simulink library "LIB_InputsProcessing"  (R2018b)
settings: Solver=VariableStepAuto  StartTime=0.0  StopTime=10.0  RelTol=1e-3
undefined symbols (not defined in the file or in its folder): rTBlowerMotorMeasuredFilter, rVBatteryMeasuredFilter, TBlowerMotorScaledValueMap, VAnalogInputSpan, VTBlowerMotorScaledValueAxis
libraries: RespiratorCtrlLib x11
settings Model: Creator=BRAUL  LastModifiedBy=VITIE

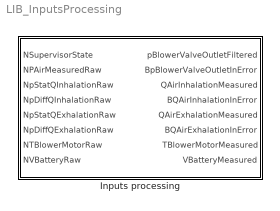
== system LIB_InputsProcessing ==
  Inputs processing : Subsystem
      settings: AttributesFormatString=%<ReferenceBlock>

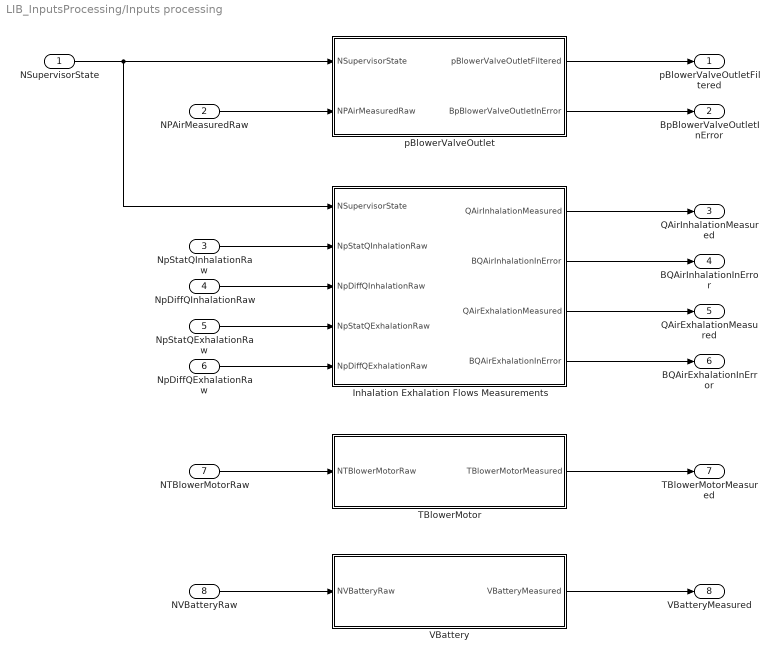
== system LIB_InputsProcessing/Inputs processing ==
  NSupervisorState : Inport  OutDataTypeStr=Enum: eSupervisorStates
  NPAirMeasuredRaw : Inport  Port=2
  NpStatQInhalationRaw : Inport  Port=3  OutDataTypeStr=single
  NpDiffQInhalationRaw : Inport  Port=4  OutDataTypeStr=single
  NpStatQExhalationRaw : Inport  Port=5  OutDataTypeStr=single
  NpDiffQExhalationRaw : Inport  Port=6  OutDataTypeStr=single
  NTBlowerMotorRaw : Inport  Port=7
  NVBatteryRaw : Inport  Port=8
  Inhalation Exhalation Flows Measurements : Subsystem
  TBlowerMotor : Subsystem
  VBattery : Subsystem
  pBlowerValveOutlet : Subsystem
  pBlowerValveOutletFiltered : Outport
  BpBlowerValveOutletInError : Outport  Port=2  OutDataTypeStr=boolean
  QAirInhalationMeasured : Outport  Port=3  OutDataTypeStr=single
  BQAirInhalationInError : Outport  Port=4  OutDataTypeStr=boolean
  QAirExhalationMeasured : Outport  Port=5  OutDataTypeStr=single
  BQAirExhalationInError : Outport  Port=6  OutDataTypeStr=boolean
  TBlowerMotorMeasured : Outport  Port=7
  VBatteryMeasured : Outport  Port=8
  wires:
  Inhalation Exhalation Flows Measurements/4(BQAirExhalationInError) -> BQAirExhalationInError/1
  Inhalation Exhalation Flows Measurements/3(QAirExhalationMeasured) -> QAirExhalationMeasured/1
  Inhalation Exhalation Flows Measurements/2(BQAirInhalationInError) -> BQAirInhalationInError/1
  Inhalation Exhalation Flows Measurements/1(QAirInhalationMeasured) -> QAirInhalationMeasured/1
  NpDiffQExhalationRaw/1 -> Inhalation Exhalation Flows Measurements/5(NpDiffQExhalationRaw)
  NpStatQExhalationRaw/1 -> Inhalation Exhalation Flows Measurements/4(NpStatQExhalationRaw)
  NpDiffQInhalationRaw/1 -> Inhalation Exhalation Flows Measurements/3(NpDiffQInhalationRaw)
  NpStatQInhalationRaw/1 -> Inhalation Exhalation Flows Measurements/2(NpStatQInhalationRaw)
  pBlowerValveOutlet/1(pBlowerValveOutletFiltered) -> pBlowerValveOutletFiltered/1
  pBlowerValveOutlet/2(BpBlowerValveOutletInError) -> BpBlowerValveOutletInError/1
  NSupervisorState/1 -> pBlowerValveOutlet/1(NSupervisorState), Inhalation Exhalation Flows Measurements/1(NSupervisorState)
  NPAirMeasuredRaw/1 -> pBlowerValveOutlet/2(NPAirMeasuredRaw)
  VBattery/1(VBatteryMeasured) -> VBatteryMeasured/1
  TBlowerMotor/1(TBlowerMotorMeasured) -> TBlowerMotorMeasured/1
  NVBatteryRaw/1 -> VBattery/1(NVBatteryRaw)
  NTBlowerMotorRaw/1 -> TBlowerMotor/1(NTBlowerMotorRaw)

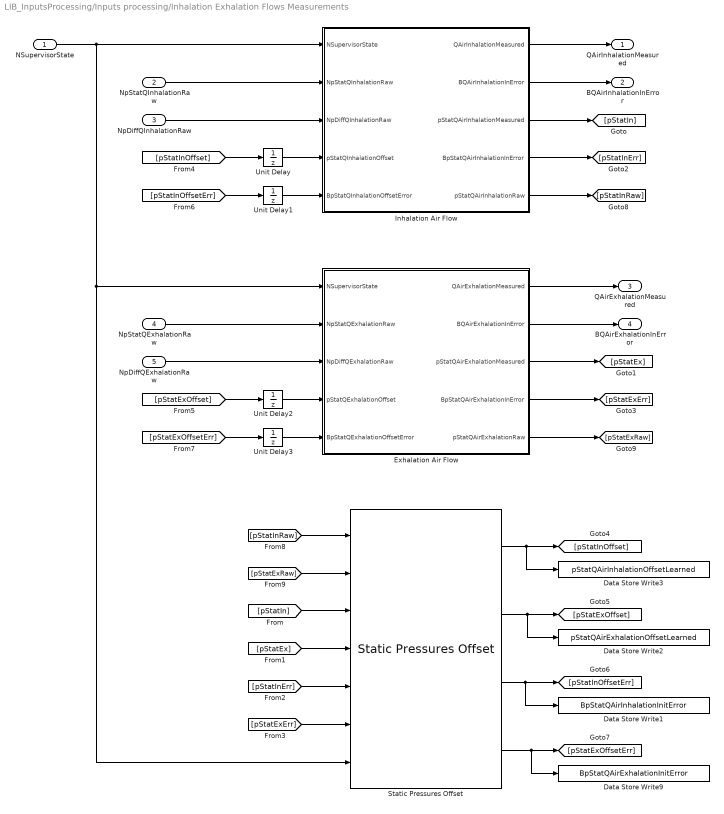
== system LIB_InputsProcessing/Inputs processing/Inhalation Exhalation Flows Measurements ==
  NSupervisorState : Inport  OutDataTypeStr=Enum: eSupervisorStates
  NpStatQInhalationRaw : Inport  Port=2  OutDataTypeStr=single
  NpDiffQInhalationRaw : Inport  Port=3  OutDataTypeStr=single
  NpStatQExhalationRaw : Inport  Port=4  OutDataTypeStr=single
  NpDiffQExhalationRaw : Inport  Port=5  OutDataTypeStr=single
  Data Store Write1 : DataStoreWrite  DataStoreName=BpStatQAirInhalationInitError
  Data Store Write2 : DataStoreWrite  DataStoreName=pStatQAirExhalationOffsetLearned
  Data Store Write3 : DataStoreWrite  DataStoreName=pStatQAirInhalationOffsetLearned
  Data Store Write9 : DataStoreWrite  DataStoreName=BpStatQAirExhalationInitError
  Exhalation Air Flow : Subsystem
  Inhalation Air Flow : Subsystem
  Static Pressures Offset : RespiratorCtrlLib/Inputs/Static Pressures Offset  pOffsetMin=pStatQAirAutoOffsetMin  pOffsetMax=pStatQAirAutoOffsetMax  pOffsetRateMax=pStatQAirAutoOffsetRateMax
  Unit Delay{,1..3} (4 alike) : UnitDelay  SampleTime=-1
  QAirInhalationMeasured : Outport  OutDataTypeStr=single
  BQAirInhalationInError : Outport  Port=2  OutDataTypeStr=boolean
  QAirExhalationMeasured : Outport  Port=3  OutDataTypeStr=single
  BQAirExhalationInError : Outport  Port=4  OutDataTypeStr=boolean
  wires:
  [pStatExRaw] -> Static Pressures Offset/2
  [pStatInRaw] -> Static Pressures Offset/1
  Exhalation Air Flow/5(pStatQAirExhalationRaw) -> [pStatExRaw]
  Inhalation Air Flow/5(pStatQAirInhalationRaw) -> [pStatInRaw]
  [pStatExOffsetErr] -> Unit Delay3/1
  [pStatExOffset] -> Unit Delay2/1
  Unit Delay3/1 -> Exhalation Air Flow/5(BpStatQExhalationOffsetError)
  Unit Delay2/1 -> Exhalation Air Flow/4(pStatQExhalationOffset)
  [pStatInOffsetErr] -> Unit Delay1/1
  [pStatInOffset] -> Unit Delay/1
  Unit Delay1/1 -> Inhalation Air Flow/5(BpStatQInhalationOffsetError)
  Unit Delay/1 -> Inhalation Air Flow/4(pStatQInhalationOffset)
  Static Pressures Offset/4 -> [pStatExOffsetErr], Data Store Write9/1
  Static Pressures Offset/3 -> [pStatInOffsetErr], Data Store Write1/1
  Static Pressures Offset/2 -> [pStatExOffset], Data Store Write2/1
  Static Pressures Offset/1 -> [pStatInOffset], Data Store Write3/1
  [pStatExErr] -> Static Pressures Offset/6
  [pStatInErr] -> Static Pressures Offset/5
  [pStatEx] -> Static Pressures Offset/4
  [pStatIn] -> Static Pressures Offset/3
  Exhalation Air Flow/4(BpStatQAirExhalationInError) -> [pStatExErr]
  Inhalation Air Flow/4(BpStatQAirInhalationInError) -> [pStatInErr]
  Exhalation Air Flow/3(pStatQAirExhalationMeasured) -> [pStatEx]
  Inhalation Air Flow/3(pStatQAirInhalationMeasured) -> [pStatIn]
  NSupervisorState/1 -> Exhalation Air Flow/1(NSupervisorState), Static Pressures Offset/7, Inhalation Air Flow/1(NSupervisorState)
  Exhalation Air Flow/2(BQAirExhalationInError) -> BQAirExhalationInError/1
  Exhalation Air Flow/1(QAirExhalationMeasured) -> QAirExhalationMeasured/1
  Inhalation Air Flow/2(BQAirInhalationInError) -> BQAirInhalationInError/1
  Inhalation Air Flow/1(QAirInhalationMeasured) -> QAirInhalationMeasured/1
  NpDiffQExhalationRaw/1 -> Exhalation Air Flow/3(NpDiffQExhalationRaw)
  NpStatQExhalationRaw/1 -> Exhalation Air Flow/2(NpStatQExhalationRaw)
  NpDiffQInhalationRaw/1 -> Inhalation Air Flow/3(NpDiffQInhalationRaw)
  NpStatQInhalationRaw/1 -> Inhalation Air Flow/2(NpStatQInhalationRaw)

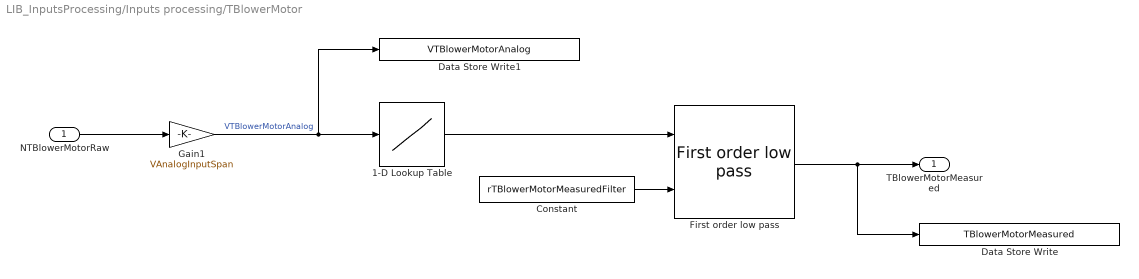
== system LIB_InputsProcessing/Inputs processing/TBlowerMotor ==
  NTBlowerMotorRaw : Inport
  1-D Lookup Table : Lookup_n-D  NumberOfTableDimensions=1  BreakpointsForDimension1=VTBlowerMotorScaledValueAxis  BeginIndexSearchUsingPreviousIndexResult=on  Table=TBlowerMotorScaledValueMap  ExtrapMethod=Clip  RemoveProtectionInput=on  UseLastTableValue=on  InternalRulePriority=Speed  RndMeth=Simplest  InputSameDT=on
  Constant : Constant  Value=rTBlowerMotorMeasuredFilter
  Data Store Write : DataStoreWrite  DataStoreName=TBlowerMotorMeasured
  Data Store Write1 : DataStoreWrite  DataStoreName=VTBlowerMotorAnalog
  First order low pass : RespiratorCtrlLib/Filters/First order low pass  SystemSampleTime=-1
  Gain1 : Gain  Gain=VAnalogInputSpan
      settings: AttributesFormatString=%<Gain>
  TBlowerMotorMeasured : Outport
  wires:
  Constant/1 -> First order low pass/2
  1-D Lookup Table/1 -> First order low pass/1
  Gain1/1 -> 1-D Lookup Table/1, Data Store Write1/1  "VTBlowerMotorAnalog"
  First order low pass/1 -> TBlowerMotorMeasured/1, Data Store Write/1
  NTBlowerMotorRaw/1 -> Gain1/1

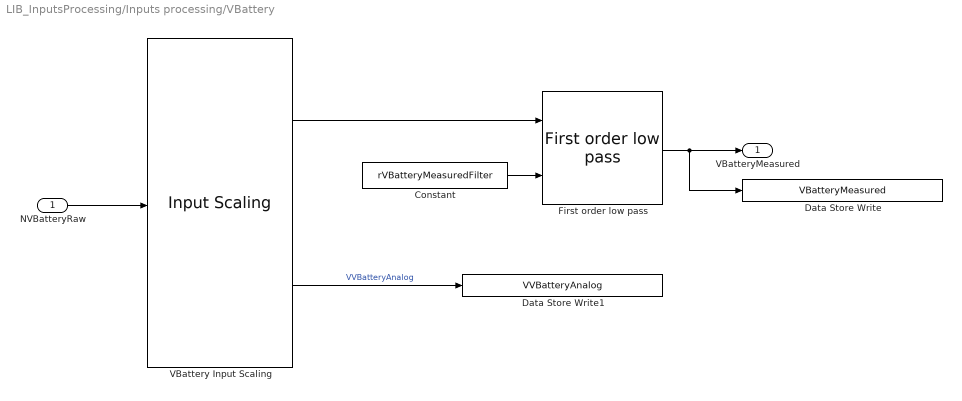
== system LIB_InputsProcessing/Inputs processing/VBattery ==
  NVBatteryRaw : Inport
  Constant : Constant  Value=rVBatteryMeasuredFilter
  Data Store Write : DataStoreWrite  DataStoreName=VBatteryMeasured
  Data Store Write1 : DataStoreWrite  DataStoreName=VVBatteryAnalog
  First order low pass : RespiratorCtrlLib/Filters/First order low pass  SystemSampleTime=-1
  VBattery Input Scaling : RespiratorCtrlLib/Inputs/Input Scaling  inputName=VBattery  elecMin=VVBatteryAnalogMin  elecMax=VVBatteryAnalogMax  physicMin=VBatteryMeasuredScaleMin  physicMax=VBatteryMeasuredScaleMax  gain=0  offset=0
  VBatteryMeasured : Outport
  wires:
  NVBatteryRaw/1 -> VBattery Input Scaling/1
  VBattery Input Scaling/2 -> Data Store Write1/1  "VVBatteryAnalog"
  First order low pass/1 -> VBatteryMeasured/1, Data Store Write/1
  VBattery Input Scaling/1 -> First order low pass/1
  Constant/1 -> First order low pass/2

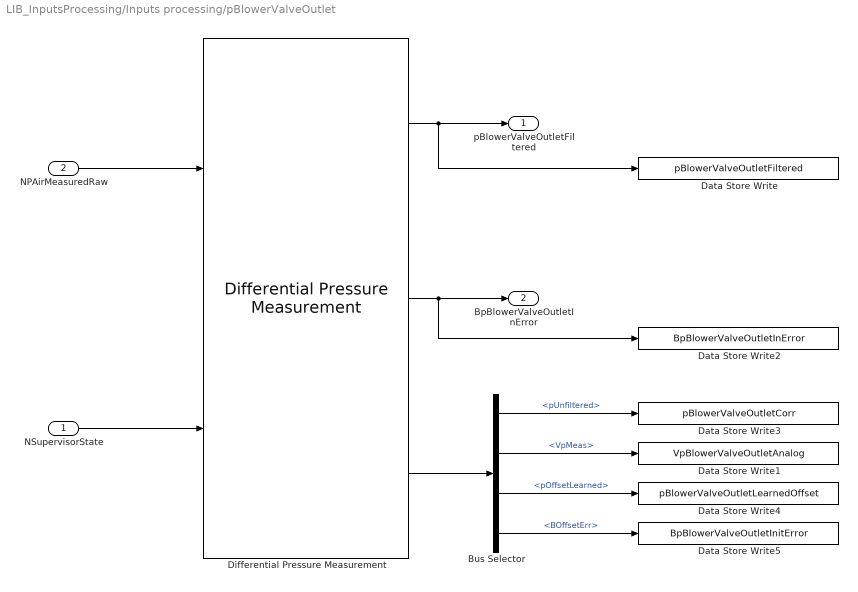
== system LIB_InputsProcessing/Inputs processing/pBlowerValveOutlet ==
  NSupervisorState : Inport  OutDataTypeStr=Enum: eSupervisorStates
  NPAirMeasuredRaw : Inport  Port=2
  Bus Selector : BusSelector  OutputSignals=pUnfiltered,VpMeas,pOffsetLearned,BOffsetErr
  Data Store Write : DataStoreWrite  DataStoreName=pBlowerValveOutletFiltered
  Data Store Write1 : DataStoreWrite  DataStoreName=VpBlowerValveOutletAnalog
  Data Store Write2 : DataStoreWrite  DataStoreName=BpBlowerValveOutletInError
  Data Store Write3 : DataStoreWrite  DataStoreName=pBlowerValveOutletCorr
  Data Store Write4 : DataStoreWrite  DataStoreName=pBlowerValveOutletLearnedOffset
  Data Store Write5 : DataStoreWrite  DataStoreName=BpBlowerValveOutletInitError
  Differential Pressure Measurement : RespiratorCtrlLib/Inputs/Differential Pressure Measurement  MeasName=pBlowerValveOutlet  AnalogMin=VpBlowerValveOutletAnalogMin  AnalogMax=VpBlowerValveOutletAnalogMax  PressureMin=pBlowerValveOutletScaledMin  PressureMax=pBlowerValveOutletScaledMax  ZeroOffset=pBlowerValveOutletMeasureOffset  CutOffFreq=fpBlowerValveOutletFilter  pOffsetMin=pBlowerValveOutletOffsetMin  pOffsetMax=pBlowerValveOutletOffsetMax  pOffsetRateMax=pBlowerValveOutletOffsetRateMax  VAnaMinDiag=VpBlowerValveOutletAnalogDiagMin  VAnaMaxDiag=VpBlowerValveOutletAnalogDiagMax
  pBlowerValveOutletFiltered : Outport
  BpBlowerValveOutletInError : Outport  Port=2  OutDataTypeStr=boolean
  wires:
  Bus Selector/4 -> Data Store Write5/1  "<BOffsetErr>"
  Bus Selector/3 -> Data Store Write4/1  "<pOffsetLearned>"
  Bus Selector/1 -> Data Store Write3/1  "<pUnfiltered>"
  Bus Selector/2 -> Data Store Write1/1  "<VpMeas>"
  Differential Pressure Measurement/3 -> Bus Selector/1
  NSupervisorState/1 -> Differential Pressure Measurement/2
  NPAirMeasuredRaw/1 -> Differential Pressure Measurement/1
  Differential Pressure Measurement/2 -> BpBlowerValveOutletInError/1, Data Store Write2/1
  Differential Pressure Measurement/1 -> pBlowerValveOutletFiltered/1, Data Store Write/1

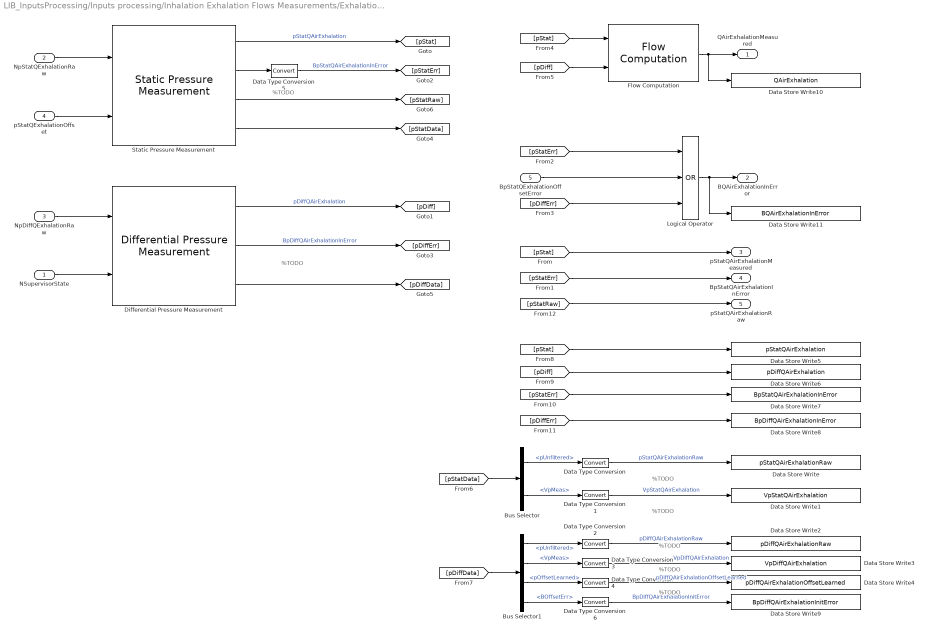
== system LIB_InputsProcessing/Inputs processing/Inhalation Exhalation Flows Measurements/Exhalation Air Flow ==
  note: %TODO
  note: %TODO
  note: %TODO
  note: %TODO
  note: %TODO
  note: %TODO
  note: %TODO
  NSupervisorState : Inport  OutDataTypeStr=Enum: eSupervisorStates
  NpStatQExhalationRaw : Inport  Port=2  OutDataTypeStr=single
  NpDiffQExhalationRaw : Inport  Port=3  OutDataTypeStr=single
  pStatQExhalationOffset : Inport  Port=4  OutDataTypeStr=single
  BpStatQExhalationOffsetError : Inport  Port=5  OutDataTypeStr=boolean
  Bus Selector : BusSelector  OutputSignals=pUnfiltered,VpMeas
  Bus Selector1 : BusSelector  OutputSignals=pUnfiltered,VpMeas,pOffsetLearned,BOffsetErr
  Data Store Write : DataStoreWrite  DataStoreName=pStatQAirExhalationRaw
  Data Store Write1 : DataStoreWrite  DataStoreName=VpStatQAirExhalation
  Data Store Write10 : DataStoreWrite  DataStoreName=QAirExhalation
  Data Store Write11 : DataStoreWrite  DataStoreName=BQAirExhalationInError
  Data Store Write2 : DataStoreWrite  DataStoreName=pDiffQAirExhalationRaw
  Data Store Write3 : DataStoreWrite  DataStoreName=VpDiffQAirExhalation
  Data Store Write4 : DataStoreWrite  DataStoreName=pDiffQAirExhalationOffsetLearned
  Data Store Write5 : DataStoreWrite  DataStoreName=pStatQAirExhalation
  Data Store Write6 : DataStoreWrite  DataStoreName=pDiffQAirExhalation
  Data Store Write7 : DataStoreWrite  DataStoreName=BpStatQAirExhalationInError
  Data Store Write8 : DataStoreWrite  DataStoreName=BpDiffQAirExhalationInError
  Data Store Write9 : DataStoreWrite  DataStoreName=BpDiffQAirExhalationInitError
  Data Type Conversion{,1..6} (7 alike) : DataTypeConversion
  Differential Pressure Measurement : RespiratorCtrlLib/Inputs/Differential Pressure Measurement  MeasName=Exhalation differential pressure  AnalogMin=VpDiffQAirAnalogicMin  AnalogMax=VpDiffQAirAnalogicMax  PressureMin=pDiffQAirScaledMax  PressureMax=pDiffQAirScaledMin  ZeroOffset=pDiffQAirExhalationOffset  CutOffFreq=fpDiffQAirExhalation  pOffsetMin=pDiffQAirAutoOffsetMin  pOffsetMax=pDiffQAirAutoOffsetMax  pOffsetRateMax=pDiffQAirAutoOffsetRateMax  VAnaMinDiag=VpDiffQAirAnalogicDiagMin  VAnaMaxDiag=VpDiffQAirAnalogicDiagMax
  Flow Computation : RespiratorCtrlLib/Inputs/Flow Computation  measName=Exhalation  QRef=QExhalationReference  PStatRef=pStaticQExhalationReference  PDiffRef=pDifferentialQExhalationReference  kAlpha=kAlphaQExhalation  kBeta=kBetaQExhalation
  Logical Operator : Logic  Operator=OR  Inputs=3  AllPortsSameDT=off  OutDataTypeStr=boolean
  Static Pressure Measurement : RespiratorCtrlLib/Inputs/Static Pressure Measurement  MeasName=Exhalation static pressure  AnalogMin=VpStatQAirAnalogicMin  AnalogMax=VpStatQAirAnalogicMax  PressureMin=pStatQAirScaledMin  PressureMax=pStatQAirScaledMax  ZeroOffset=pStatQAirExhalationOffset  CutOffFreq=fpStatQAirExhalation  VAnaMinDiag=VpStatQAirAnalogicDiagMin  VAnaMaxDiag=VpStatQAirAnalogicDiagMax
  QAirExhalationMeasured : Outport  OutDataTypeStr=single
  BQAirExhalationInError : Outport  Port=2  OutDataTypeStr=boolean
  pStatQAirExhalationMeasured : Outport  Port=3  OutDataTypeStr=single
  BpStatQAirExhalationInError : Outport  Port=4  OutDataTypeStr=boolean
  pStatQAirExhalationRaw : Outport  Port=5  OutDataTypeStr=single
  wires:
  [pStatRaw] -> pStatQAirExhalationRaw/1
  Static Pressure Measurement/3 -> [pStatRaw]
  Static Pressure Measurement/4 -> [pStatData]
  Data Type Conversion6/1 -> Data Store Write9/1  "BpDiffQAirExhalationInitError"
  Bus Selector1/4 -> Data Type Conversion6/1  "<BOffsetErr>"
  Data Type Conversion5/1 -> [pStatErr]  "BpStatQAirExhalationInError"
  [pStatData] -> Bus Selector/1
  [pDiffData] -> Bus Selector1/1
  Bus Selector/1 -> Data Type Conversion/1  "<pUnfiltered>"
  Bus Selector/2 -> Data Type Conversion1/1  "<VpMeas>"
  Bus Selector1/1 -> Data Type Conversion2/1  "<pUnfiltered>"
  Bus Selector1/2 -> Data Type Conversion3/1  "<VpMeas>"
  Bus Selector1/3 -> Data Type Conversion4/1  "<pOffsetLearned>"
  Data Type Conversion/1 -> Data Store Write/1  "pStatQAirExhalationRaw"
  Data Type Conversion1/1 -> Data Store Write1/1  "VpStatQAirExhalation"
  Data Type Conversion2/1 -> Data Store Write2/1  "pDiffQAirExhalationRaw"
  Data Type Conversion3/1 -> Data Store Write3/1  "VpDiffQAirExhalation"
  Data Type Conversion4/1 -> Data Store Write4/1  "pDiffQAirExhalationOffsetLearned"
  [pStat] -> Data Store Write5/1
  [pDiff] -> Data Store Write6/1
  [pStatErr] -> Data Store Write7/1
  [pDiffErr] -> Data Store Write8/1
  NSupervisorState/1 -> Differential Pressure Measurement/2
  NpDiffQExhalationRaw/1 -> Differential Pressure Measurement/1
  pStatQExhalationOffset/1 -> Static Pressure Measurement/2
  NpStatQExhalationRaw/1 -> Static Pressure Measurement/1
  [pDiffErr] -> Logical Operator/3
  Differential Pressure Measurement/3 -> [pDiffData]
  Differential Pressure Measurement/1 -> [pDiff]  "pDiffQAirExhalation"
  Static Pressure Measurement/1 -> [pStat]  "pStatQAirExhalation"
  Differential Pressure Measurement/2 -> [pDiffErr]  "BpDiffQAirExhalationInError"
  [pStatErr] -> Logical Operator/1
  Logical Operator/1 -> BQAirExhalationInError/1, Data Store Write11/1
  [pStat] -> pStatQAirExhalationMeasured/1
  BpStatQExhalationOffsetError/1 -> Logical Operator/2
  [pStat] -> Flow Computation/1
  Flow Computation/1 -> QAirExhalationMeasured/1, Data Store Write10/1
  [pDiff] -> Flow Computation/2
  Static Pressure Measurement/2 -> Data Type Conversion5/1
  [pStatErr] -> BpStatQAirExhalationInError/1

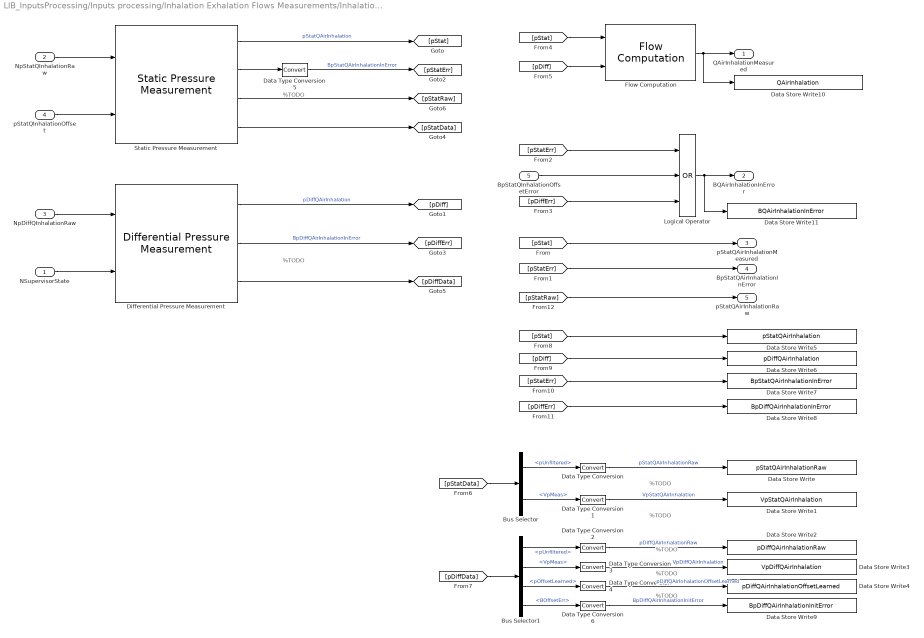
== system LIB_InputsProcessing/Inputs processing/Inhalation Exhalation Flows Measurements/Inhalation Air Flow ==
  note: %TODO
  note: %TODO
  note: %TODO
  note: %TODO
  note: %TODO
  note: %TODO
  note: %TODO
  NSupervisorState : Inport  OutDataTypeStr=Enum: eSupervisorStates
  NpStatQInhalationRaw : Inport  Port=2  OutDataTypeStr=single
  NpDiffQInhalationRaw : Inport  Port=3  OutDataTypeStr=single
  pStatQInhalationOffset : Inport  Port=4  OutDataTypeStr=single
  BpStatQInhalationOffsetError : Inport  Port=5  OutDataTypeStr=boolean
  Bus Selector : BusSelector  OutputSignals=pUnfiltered,VpMeas
  Bus Selector1 : BusSelector  OutputSignals=pUnfiltered,VpMeas,pOffsetLearned,BOffsetErr
  Data Store Write : DataStoreWrite  DataStoreName=pStatQAirInhalationRaw
  Data Store Write1 : DataStoreWrite  DataStoreName=VpStatQAirInhalation
  Data Store Write10 : DataStoreWrite  DataStoreName=QAirInhalation
  Data Store Write11 : DataStoreWrite  DataStoreName=BQAirInhalationInError
  Data Store Write2 : DataStoreWrite  DataStoreName=pDiffQAirInhalationRaw
  Data Store Write3 : DataStoreWrite  DataStoreName=VpDiffQAirInhalation
  Data Store Write4 : DataStoreWrite  DataStoreName=pDiffQAirInhalationOffsetLearned
  Data Store Write5 : DataStoreWrite  DataStoreName=pStatQAirInhalation
  Data Store Write6 : DataStoreWrite  DataStoreName=pDiffQAirInhalation
  Data Store Write7 : DataStoreWrite  DataStoreName=BpStatQAirInhalationInError
  Data Store Write8 : DataStoreWrite  DataStoreName=BpDiffQAirInhalationInError
  Data Store Write9 : DataStoreWrite  DataStoreName=BpDiffQAirInhalationInitError
  Data Type Conversion{,1..6} (7 alike) : DataTypeConversion
  Differential Pressure Measurement : RespiratorCtrlLib/Inputs/Differential Pressure Measurement  MeasName=Inhalation differential pressure  AnalogMin=VpDiffQAirAnalogicMin  AnalogMax=VpDiffQAirAnalogicMax  PressureMin=pDiffQAirScaledMax  PressureMax=pDiffQAirScaledMin  ZeroOffset=pDiffQAirInhalationOffset  CutOffFreq=fpDiffQAirInhalation  pOffsetMin=pDiffQAirAutoOffsetMin  pOffsetMax=pDiffQAirAutoOffsetMax  pOffsetRateMax=pDiffQAirAutoOffsetRateMax  VAnaMinDiag=VpDiffQAirAnalogicDiagMin  VAnaMaxDiag=VpDiffQAirAnalogicDiagMax
  Flow Computation : RespiratorCtrlLib/Inputs/Flow Computation  measName=Inhalation  QRef=QInhalationReference  PStatRef=pStaticQInhalationReference  PDiffRef=pDifferentialQInhalationReference  kAlpha=kAlphaQInhalation  kBeta=kBetaQInhalation
  Logical Operator : Logic  Operator=OR  Inputs=3  AllPortsSameDT=off  OutDataTypeStr=boolean
  Static Pressure Measurement : RespiratorCtrlLib/Inputs/Static Pressure Measurement  MeasName=Inhalation static pressure  AnalogMin=VpStatQAirAnalogicMin  AnalogMax=VpStatQAirAnalogicMax  PressureMin=pStatQAirScaledMin  PressureMax=pStatQAirScaledMax  ZeroOffset=pStatQAirInhalationOffset  CutOffFreq=fpStatQAirInhalation  VAnaMinDiag=VpStatQAirAnalogicDiagMin  VAnaMaxDiag=VpStatQAirAnalogicDiagMax
  QAirInhalationMeasured : Outport  OutDataTypeStr=single
  BQAirInhalationInError : Outport  Port=2  OutDataTypeStr=boolean
  pStatQAirInhalationMeasured : Outport  Port=3  OutDataTypeStr=single
  BpStatQAirInhalationInError : Outport  Port=4  OutDataTypeStr=boolean
  pStatQAirInhalationRaw : Outport  Port=5  OutDataTypeStr=single
  wires:
  [pStatRaw] -> pStatQAirInhalationRaw/1
  Static Pressure Measurement/3 -> [pStatRaw]
  Data Type Conversion6/1 -> Data Store Write9/1  "BpDiffQAirInhalationInitError"
  Bus Selector1/4 -> Data Type Conversion6/1  "<BOffsetErr>"
  Data Type Conversion5/1 -> [pStatErr]  "BpStatQAirInhalationInError"
  [pDiffErr] -> Data Store Write8/1
  [pStatErr] -> Data Store Write7/1
  [pDiff] -> Data Store Write6/1
  [pStat] -> Data Store Write5/1
  Data Type Conversion4/1 -> Data Store Write4/1  "pDiffQAirInhalationOffsetLearned"
  Data Type Conversion3/1 -> Data Store Write3/1  "VpDiffQAirInhalation"
  Data Type Conversion2/1 -> Data Store Write2/1  "pDiffQAirInhalationRaw"
  Data Type Conversion1/1 -> Data Store Write1/1  "VpStatQAirInhalation"
  Data Type Conversion/1 -> Data Store Write/1  "pStatQAirInhalationRaw"
  Bus Selector1/3 -> Data Type Conversion4/1  "<pOffsetLearned>"
  Bus Selector1/2 -> Data Type Conversion3/1  "<VpMeas>"
  Bus Selector1/1 -> Data Type Conversion2/1  "<pUnfiltered>"
  Bus Selector/2 -> Data Type Conversion1/1  "<VpMeas>"
  Bus Selector/1 -> Data Type Conversion/1  "<pUnfiltered>"
  [pDiffData] -> Bus Selector1/1
  [pStatData] -> Bus Selector/1
  [pDiff] -> Flow Computation/2
  [pStat] -> Flow Computation/1
  Flow Computation/1 -> QAirInhalationMeasured/1, Data Store Write10/1
  [pDiffErr] -> Logical Operator/3
  BpStatQInhalationOffsetError/1 -> Logical Operator/2
  [pStatErr] -> Logical Operator/1
  Logical Operator/1 -> BQAirInhalationInError/1, Data Store Write11/1
  [pStat] -> pStatQAirInhalationMeasured/1
  [pStatErr] -> BpStatQAirInhalationInError/1
  Differential Pressure Measurement/3 -> [pDiffData]
  Static Pressure Measurement/4 -> [pStatData]
  Differential Pressure Measurement/2 -> [pDiffErr]  "BpDiffQAirInhalationInError"
  Static Pressure Measurement/2 -> Data Type Conversion5/1
  Differential Pressure Measurement/1 -> [pDiff]  "pDiffQAirInhalation"
  Static Pressure Measurement/1 -> [pStat]  "pStatQAirInhalation"
  NSupervisorState/1 -> Differential Pressure Measurement/2
  NpDiffQInhalationRaw/1 -> Differential Pressure Measurement/1
  pStatQInhalationOffset/1 -> Static Pressure Measurement/2
  NpStatQInhalationRaw/1 -> Static Pressure Measurement/1
